simulink model "controller_velocity_north"  (R2021a)
settings: Solver=FixedStepAuto  StartTime=0.0  StopTime=10.0  FixedStep=0.002  RelTol=1e-3
undefined symbols (not defined in the file): DiscIntNeverNeededParam, G_VN_OL_DENOM, G_VN_OL_NUM, K_ud, K_ui, K_up, max_vel_xy, vel_dterm_cutoff, vel_filt_denom, vel_filt_num
libraries: simulink x1, pid_lib x1
settings Model: Creator=francois  LastModifiedBy=esl
settings SolverCC: AlgebraicLoopSolver=TrustRegion
settings DebuggingCC: SFMachineParentedDataDiag=warning

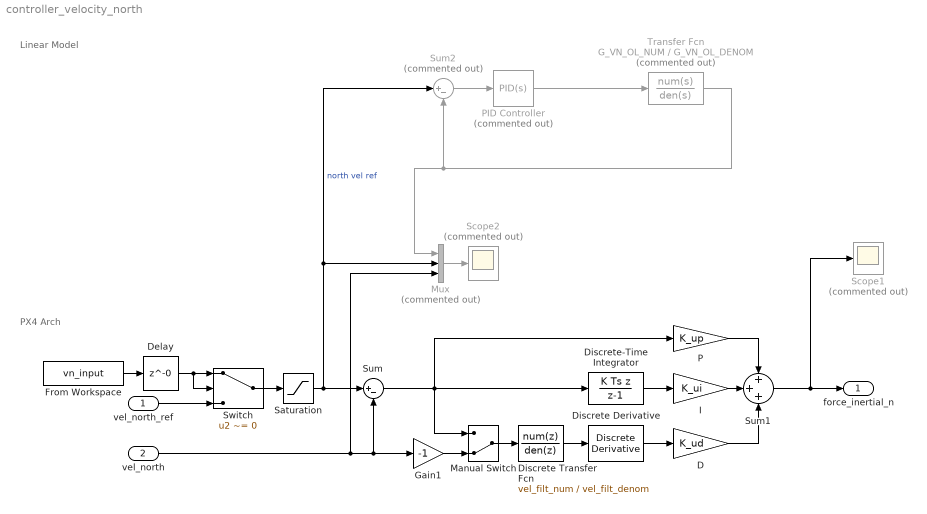
== system controller_velocity_north ==
  note: Linear Model
  note: PX4 Arch
  vel_north_ref : Inport
  vel_north : Inport  Port=2
  D : Gain  Gain=K_ud
  Delay : Delay  DelayLength=0
  Discrete Transfer Fcn : DiscreteTransferFcn  Numerator=vel_filt_num  Denominator=vel_filt_denom
  Discrete Derivative : simulink/Discrete/Discrete Derivative  gainval=1  ICPrevScaledInput=0.0  OutMin=[]  OutMax=[]  OutDataType=fixdt(1, 16)  OutScaling=2^-10  DoSatur=off
  Discrete-Time Integrator : DiscreteIntegrator  IntegratorMethod=Integration: Backward Euler  gainval=1  SampleTime=-1  UpperSaturationLimit=max_vel_xy  LowerSaturationLimit=-max_vel_xy  ICPrevOutput=DiscIntNeverNeededParam  ICPrevScaledInput=DiscIntNeverNeededParam
  From Workspace : FromWorkspace  VariableName=vn_input
  Gain1 : Gain  Gain=-1
  I : Gain  Gain=K_ui
  Manual Switch : ManualSwitch  CurrentSetting=0
  Mux : Mux  Commented=on  Inputs=3
  P : Gain  Gain=K_up
  PID Controller : pid_lib/PID Controller  Commented=on  Controller=PID  Form=Parallel  TimeDomain=Continuous-time  UseExternalTs=off  SampleTime=-1  IntegratorMethod=Forward Euler  FilterMethod=Forward Euler  ControllerParametersSource=internal  P=K_up  I=K_ui  D=K_ud  UseFilter=on  N=vel_dterm_cutoff*10  TunerSelectOption=Transfer Function Based (PID Tuner App)  InitialConditionSource=internal  InitialConditionForIntegrator=0  InitialConditionForFilter=0  DifferentiatorICPrevScaledInput=0  ExternalReset=none  TrackingMode=off  Kt=1  LimitOutput=off  SatLimitsSource=internal  UpperSaturationLimit=inf  LowerSaturationLimit=-inf  LinearizeAsGain=on  AntiWindupMode=none  Kb=1  POutMin=[]  POutMax=[]  IOutMin=[]  IOutMax=[]  DOutMin=[]  DOutMax=[]  NOutMin=[]  NOutMax=[]  SumOutMin=[]  SumOutMax=[]  SaturationOutMin=[]  SaturationOutMax=[]  PParamMin=[]  PParamMax=[]  IParamMin=[]  IParamMax=[]  DParamMin=[]  DParamMax=[]  NParamMin=[]  NParamMax=[]  KbParamMin=[]  KbParamMax=[]  KtParamMin=[]  KtParamMax=[]  KbOutMin=[]  KbOutMax=[]  KtOutMin=[]  KtOutMax=[]  IntegratorOutMin=[]  IntegratorOutMax=[]  FilterOutMin=[]  FilterOutMax=[]  SumI1OutMin=[]  SumI1OutMax=[]  SumI2OutMin=[]  SumI2OutMax=[]  SumI3OutMin=[]  SumI3OutMax=[]  SumI4OutMin=[]  SumI4OutMax=[]  SumDOutMin=[]  SumDOutMax=[]  DifferentiatorOutMin=[]  DifferentiatorOutMax=[]  FilterDiffOutCoefMin=[]  FilterDiffOutCoefMax=[]  ReciprocalOutMin=[]  ReciprocalOutMax=[]  SumDenOutMin=[]  SumDenOutMax=[]  SumNumOutMin=[]  SumNumOutMax=[]  DivideOutMin=[]  DivideOutMax=[]  UdiffTsProdOutMin=[]  UdiffTsProdOutMax=[]  NTsProdOutMin=[]  NTsProdOutMax=[]  UintegralTsProdOutMin=[]  UintegralTsProdOutMax=[]  UngainTsProdOutMin=[]  UngainTsProdOutMax=[]  IntegratorContinuousStateAttributes=''  IntegratorStateMustResolveToSignalObject=off  IntegratorRTWStateStorageClass=Auto  FilterContinuousStateAttributes=''  FilterStateMustResolveToSignalObject=off  FilterRTWStateStorageClass=Auto  ParallelPVariant=InternalParameters  IdealPVariant=Disabled  IVariant=InternalParameters  DVariant=InternalParameters  IntegratorVariant=Continuous  SatVariant=Disabled  AWVariant=Passthrough  PCopyVariant=Disabled  TRVariant=Disabled  FdbkBlocksVariant=Forward  IdealPFdbkVariant=Disabled  SatFdbkVariant=Disabled  DerivativeFilterVariant=ContFilter  NVariant=InternalParameters  NCopyVariant=Disabled  FilterICVariant=InternalICsFilter  IntegratorICVariant=InternalICs  ExternalResetVariant=Disabled  TRSumVariant=Passthrough  SumFdbkVariant=Disabled  SumVariant=Sum_PID  TsampFilterVariant=InternalTs  TsampNgainVariant=Passthrough  TsampIntegralVariant=Passthrough  ExternalSaturationOutDataTypeStr=Inherit: Same as second input
  Saturation : Saturate  UpperLimit=max_vel_xy  LowerLimit=-max_vel_xy
  Scope1 : Scope  Commented=on
  Scope2 : Scope  Commented=on
  Sum : Sum  Inputs=|+-
  Sum1 : Sum  Inputs=+++
  Sum2 : Sum  Commented=on  Inputs=|+-
  Switch : Switch  Criteria=u2 ~= 0
  Transfer Fcn : TransferFcn  Commented=on  Numerator=G_VN_OL_NUM  Denominator=G_VN_OL_DENOM
  force_inertial_n : Outport  VectorParamsAs1DForOutWhenUnconnected=off
  wires:
  Gain1/1 -> Manual Switch/2
  vel_north_ref/1 -> Switch/3
  PID Controller/1 -> Transfer Fcn/1
  From Workspace/1 -> Delay/1
  Saturation/1 -> Sum/1, Sum2/1, Mux/2  "north vel ref"
  Manual Switch/1 -> Discrete Transfer Fcn/1
  vel_north/1 -> Mux/3, Gain1/1, Sum/2
  Sum/1 -> Manual Switch/1, Discrete-Time Integrator/1, P/1
  Discrete Transfer Fcn/1 -> Discrete Derivative/1
  Switch/1 -> Saturation/1
  Discrete-Time Integrator/1 -> I/1
  Sum2/1 -> PID Controller/1
  D/1 -> Sum1/3
  Sum1/1 -> force_inertial_n/1, Scope1/1
  Transfer Fcn/1 -> Mux/1, Sum2/2
  Discrete Derivative/1 -> D/1
  Delay/1 -> Switch/2, Switch/1
  P/1 -> Sum1/1
  I/1 -> Sum1/2
  Mux/1 -> Scope2/1
